simulink subsystem "FCS"  (R2025a)
settings: Solver=VariableStepAuto  StartTime=0.0  StopTime=10.0  RelTol=1e-3
settings Model: Creator=gurt1  LastModifiedBy=gurt1
settings RTWCC: GPUComputeCapability=3.5

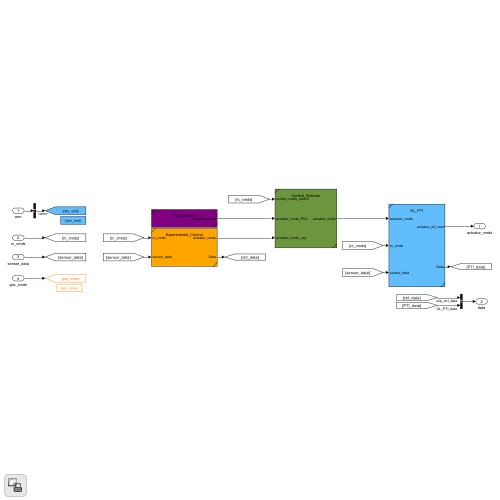
[thumbnail: Simulink's stored preview of the top-level diagram]
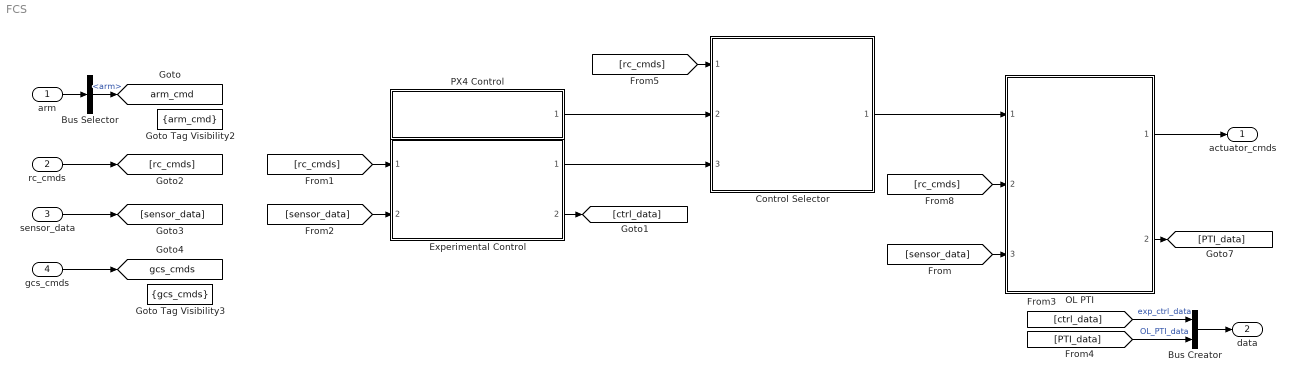
== system FCS ==
  arm : Inport
  rc_cmds : Inport  Port=2
  sensor_data : Inport  Port=3
  gcs_cmds : Inport  Port=4
  Bus Creator : BusCreator  Inputs=2
  Bus Selector : BusSelector  OutputSignals=arm
  Control Selector : Subsystem  ReferencedSubsystem=Control_Selector
  Experimental Control : Subsystem  ReferencedSubsystem=Experimental_Control
  Goto Tag Visibility2 : GotoTagVisibility  GotoTag=arm_cmd
  Goto Tag Visibility3 : GotoTagVisibility  GotoTag=gcs_cmds
  OL PTI : Subsystem  ReferencedSubsystem=OL_PTI
  PX4 Control : Subsystem  ReferencedSubsystem=PX4_Control
  actuator_cmds : Outport
  data : Outport  Port=2
  tag scope: arm_cmd=global, gcs_cmds=global
  wires:
  Bus Creator/1 -> data/1
  rc_cmds/1 -> [rc_cmds]
  sensor_data/1 -> [sensor_data]
  gcs_cmds/1 -> [gcs_cmds]
  [rc_cmds] -> OL PTI/2
  [ctrl_data] -> Bus Creator/1  "exp_ctrl_data"
  OL PTI/2 -> [PTI_data]
  [rc_cmds] -> Experimental Control/1
  [sensor_data] -> Experimental Control/2
  Control Selector/1 -> OL PTI/1
  [PTI_data] -> Bus Creator/2  "OL_PTI_data"
  arm/1 -> Bus Selector/1
  Bus Selector/1 -> [arm_cmd]  "<arm>"
  Experimental Control/2 -> [ctrl_data]
  OL PTI/1 -> actuator_cmds/1
  [sensor_data] -> OL PTI/3
  [rc_cmds] -> Control Selector/1
  PX4 Control/1 -> Control Selector/2
  Experimental Control/1 -> Control Selector/3
